simulink model "AEBS_A3X"  (Simulink 7.9)
settings: Solver=ode45  StartTime=0.0  StopTime=10.0  RelTol=1e-3
libraries: simulink x12
settings Model: Creator=fpt  LastModifiedBy=a55
settings HardwareCC: TargetIntDivRoundTo=Zero  TargetEndianess=LittleEndian  TargetHWDeviceType=MATLAB Host  ProdEqTarget=off
settings RTWCC: SystemTargetFile=rtwsfcnfmi.tlc  TemplateMakefile=rtwsfcnfmi_tmf  Description=S-function Target with Functional Model Interface (FMI)  ProcessScript=rtwsfcnfmi_make_rtw_hook
settings STFCustomTargetCC: CodeReplacementLibrary=ANSI_C  ModelReferenceCompliant=off  CompOptLevelCompliant=on  GeneratePreprocessorConditionals=Disable all  SystemTargetFile=rtwsfcnfmi.tlc
settings CustomProperty: Value=on

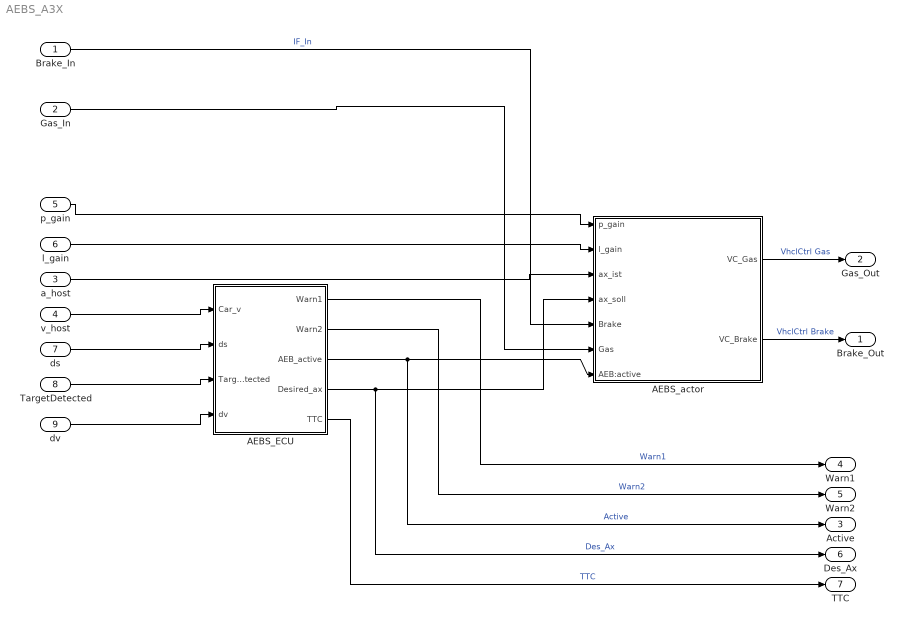
== system AEBS_A3X ==
  Brake_In : Inport  OutDataTypeStr=double
  Gas_In : Inport  Port=2  OutDataTypeStr=double
  a_host : Inport  Port=3  OutDataTypeStr=double
  v_host : Inport  Port=4  OutDataTypeStr=double
  p_gain : Inport  Port=5  OutDataTypeStr=double
  l_gain : Inport  Port=6  OutDataTypeStr=double
  ds : Inport  Port=7  OutDataTypeStr=double
  TargetDetected : Inport  Port=8  OutDataTypeStr=double
  dv : Inport  Port=9  OutDataTypeStr=double
  AEBS_ECU : Subsystem  Description=|
      | SL_REQ_010                                              
      | << Autonomous Emergency Braking ECU controller model>>
      | REQ_AB_01                    
      | R-0000057
  AEBS_actor : Subsystem  Description=|
      | SL_REQ_020                                              
      | << The Cruise control Speed Limit shall be implemented>>
      | REQ_AB_02                    
      | R-0000044                    
      | R-0000058                  
      | R-0000045
  Brake_Out : Outport  OutDataTypeStr=double
  Gas_Out : Outport  Port=2  OutDataTypeStr=double
  Active : Outport  Port=3  OutDataTypeStr=double
  Warn1 : Outport  Port=4  OutDataTypeStr=double
  Warn2 : Outport  Port=5  OutDataTypeStr=double
  Des_Ax : Outport  Port=6  OutDataTypeStr=double
  TTC : Outport  Port=7  OutDataTypeStr=double
  wires:
  AEBS_ECU/5(TTC) -> TTC/1  "TTC"
  AEBS_ECU/1(Warn1) -> Warn1/1  "Warn1"
  AEBS_ECU/2(Warn2) -> Warn2/1  "Warn2"
  AEBS_ECU/3(AEB_active) -> AEBS_actor/7(AEB:active), Active/1  "Active"
  AEBS_ECU/4(Desired_ax) -> AEBS_actor/4(ax_soll), Des_Ax/1  "Des_Ax"
  ds/1 -> AEBS_ECU/2(ds)
  v_host/1 -> AEBS_ECU/1(Car_v)
  a_host/1 -> AEBS_actor/3(ax_ist)
  p_gain/1 -> AEBS_actor/1(p_gain)
  Gas_In/1 -> AEBS_actor/6(Gas)
  TargetDetected/1 -> AEBS_ECU/3(TargetDetected)
  dv/1 -> AEBS_ECU/4(dv)
  l_gain/1 -> AEBS_actor/2(l_gain)
  Brake_In/1 -> AEBS_actor/5(Brake)  "IF_In"
  AEBS_actor/1(VC_Gas) -> Gas_Out/1  "VhclCtrl Gas"
  AEBS_actor/2(VC_Brake) -> Brake_Out/1  "VhclCtrl Brake"

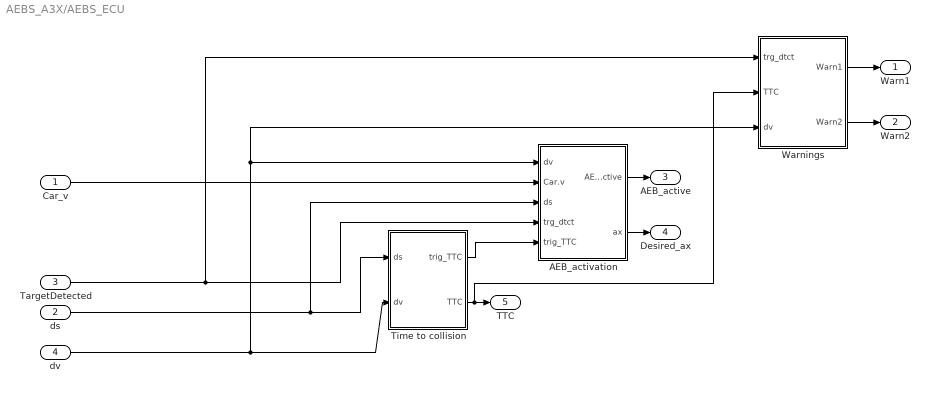
== system AEBS_A3X/AEBS_ECU ==
  Car_v : Inport  OutDataTypeStr=double
  ds : Inport  Port=2  OutDataTypeStr=double
  TargetDetected : Inport  Port=3  OutDataTypeStr=double
  dv : Inport  Port=4  OutDataTypeStr=double
  AEB_activation : Subsystem  Description=|
      | SL_REQ_011                                              
      | << The Cruise control Speed Limit shall be implemented>>
      | R-0000061                    
      | R-0000063
  Time to collision : Subsystem  Description=|
      | SL_REQ_013                                              
      | << The Cruise control Speed Limit shall be implemented>>
      | R-0000064                    
      | R-0000050                    
      | R-0000052
  Warnings : Subsystem  Description=|
      | SL_REQ_014                                              
      | << The Cruise control Speed Limit shall be implemented>>
      | R-0000048                    
      | R-0000050                    
      | R-0000052
  Warn1 : Outport  OutDataTypeStr=double
  Warn2 : Outport  Port=2  OutDataTypeStr=double
  AEB_active : Outport  Port=3  OutDataTypeStr=double
  Desired_ax : Outport  Port=4  OutDataTypeStr=double
  TTC : Outport  Port=5  OutDataTypeStr=double
  wires:
  TargetDetected/1 -> AEB_activation/4(trg_dtct), Warnings/1(trg_dtct)
  dv/1 -> AEB_activation/1(dv), Warnings/3(dv), Time to collision/2(dv)
  Time to collision/1(trig_TTC) -> AEB_activation/5(trig_TTC)
  AEB_activation/1(AEB_active) -> AEB_active/1
  Car_v/1 -> AEB_activation/2(Car.v)
  Warnings/1(Warn1) -> Warn1/1
  Warnings/2(Warn2) -> Warn2/1
  AEB_activation/2(ax) -> Desired_ax/1
  Time to collision/2(TTC) -> Warnings/2(TTC), TTC/1
  ds/1 -> AEB_activation/3(ds), Time to collision/1(ds)

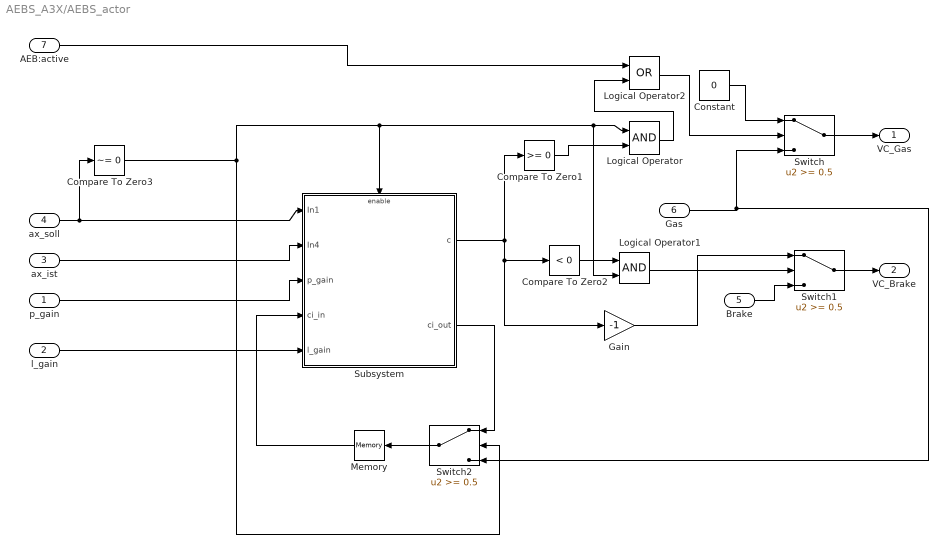
== system AEBS_A3X/AEBS_actor ==
  p_gain : Inport  OutDataTypeStr=double
  l_gain : Inport  Port=2  OutDataTypeStr=double
  ax_ist : Inport  Port=3  OutDataTypeStr=double
  ax_soll : Inport  Port=4  OutDataTypeStr=double
  Brake : Inport  Port=5  OutDataTypeStr=double
  Gas : Inport  Port=6  OutDataTypeStr=double
  AEB:active : Inport  Port=7  OutDataTypeStr=double
  Compare To Zero1 : simulink/Logic and Bit Operations/Compare To Zero  relop=>=  OutDataTypeStr=boolean
  Compare To Zero2 : simulink/Logic and Bit Operations/Compare To Zero  relop=<  OutDataTypeStr=boolean
  Compare To Zero3 : simulink/Logic and Bit Operations/Compare To Zero  relop=~=  OutDataTypeStr=boolean
  Constant : Constant  Value=0  OutDataTypeStr=double
  Gain : Gain  Gain=-1
  Logical Operator : Logic  AllPortsSameDT=off  OutDataTypeStr=boolean
  Logical Operator1 : Logic  AllPortsSameDT=off  OutDataTypeStr=boolean
  Logical Operator2 : Logic  Operator=OR  AllPortsSameDT=off  OutDataTypeStr=boolean
  Memory : Memory
  Subsystem : Subsystem
  Switch : Switch  Threshold=0.5  OutDataTypeStr=double
  Switch1 : Switch  Threshold=0.5  OutDataTypeStr=double
  Switch2 : Switch  Threshold=0.5  OutDataTypeStr=double
  VC_Gas : Outport  OutDataTypeStr=double
  VC_Brake : Outport  Port=2  OutDataTypeStr=double
  wires:
  ax_soll/1 -> Compare To Zero3/1, Subsystem/1(In1)
  ax_ist/1 -> Subsystem/2(In4)
  p_gain/1 -> Subsystem/3(p_gain)
  Switch/1 -> VC_Gas/1
  Switch1/1 -> VC_Brake/1
  Subsystem/1(c) -> Compare To Zero1/1, Compare To Zero2/1, Gain/1
  Compare To Zero1/1 -> Logical Operator/2
  Memory/1 -> Subsystem/4(ci_in)
  Subsystem/2(ci_out) -> Switch2/1
  Switch2/1 -> Memory/1
  Logical Operator1/1 -> Switch1/2
  Compare To Zero2/1 -> Logical Operator1/1
  Brake/1 -> Switch1/3
  Gain/1 -> Switch1/1
  Compare To Zero3/1 -> Logical Operator1/2, Logical Operator/1, Subsystem/Enable, Switch2/2
  Constant/1 -> Switch/1
  Gas/1 -> Switch2/3, Switch/3
  Logical Operator2/1 -> Switch/2
  Logical Operator/1 -> Logical Operator2/2
  AEB:active/1 -> Logical Operator2/1
  l_gain/1 -> Subsystem/5(l_gain)

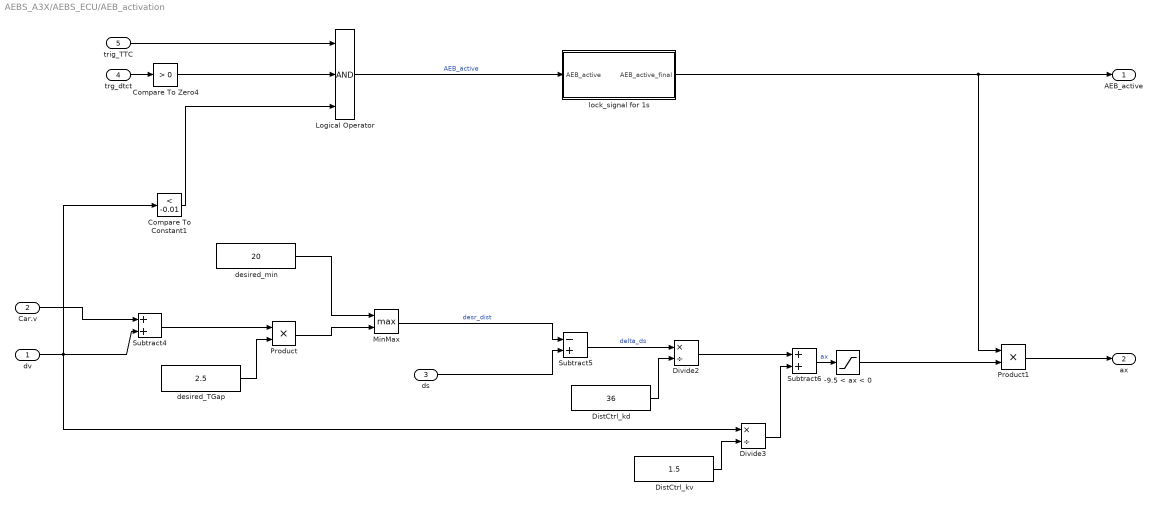
== system AEBS_A3X/AEBS_ECU/AEB_activation ==
  dv : Inport  OutDataTypeStr=double
  Car.v : Inport  Port=2  OutDataTypeStr=double
  ds : Inport  Port=3  OutDataTypeStr=double
  trg_dtct : Inport  Port=4  OutDataTypeStr=double
  trig_TTC : Inport  Description=|  Port=5  OutDataTypeStr=double
      | SL_REQ_111                                              
      | << The Cruise control Speed Limit shall be implemented>>
      | R-0000062
  -9.5 < ax < 0 : Saturate  UpperLimit=0  LowerLimit=-9.5
  Compare To Constant1 : simulink/Logic and Bit Operations/Compare To Constant  relop=<  const=-0.01  OutDataTypeStr=uint8
  Compare To Zero4 : simulink/Logic and Bit Operations/Compare To Zero  relop=>  OutDataTypeStr=uint8
  DistCtrl_kd : Constant  Value=36  OutDataTypeStr=double
  DistCtrl_kv : Constant  Value=1.5  OutDataTypeStr=double
  Divide2 : Product  Inputs=*/
  Divide3 : Product  Inputs=*/
  Logical Operator : Logic  Inputs=3  AllPortsSameDT=off  OutDataTypeStr=boolean
  MinMax : MinMax  Function=max  Inputs=2
  Product : Product  RndMeth=Zero
  Product1 : Product  RndMeth=Zero
  Subtract4 : Sum
  Subtract5 : Sum  Inputs=-+
  Subtract6 : Sum
  desired_TGap : Constant  Value=2.5  OutDataTypeStr=double
  desired_min : Constant  Value=20  OutDataTypeStr=double
  lock_signal for 1s : Subsystem  Description=|
      | SL_REQ_012                                              
      | << The Cruise control Speed Limit shall be implemented>>
      | R-0000062                  
      | R-0000050                    
      | R-0000052
  AEB_active : Outport  OutDataTypeStr=double
  ax : Outport  Port=2  OutDataTypeStr=double
  wires:
  dv/1 -> Subtract4/2, Divide3/1, Compare To Constant1/1
  Car.v/1 -> Subtract4/1
  desired_min/1 -> MinMax/1
  Subtract4/1 -> Product/1
  desired_TGap/1 -> Product/2
  Product/1 -> MinMax/2
  MinMax/1 -> Subtract5/1  "desr_dist"
  ds/1 -> Subtract5/2
  Subtract5/1 -> Divide2/1  "delta_ds"
  DistCtrl_kd/1 -> Divide2/2
  DistCtrl_kv/1 -> Divide3/2
  Divide2/1 -> Subtract6/1
  Divide3/1 -> Subtract6/2
  Subtract6/1 -> -9.5 < ax < 0/1  "ax"
  trg_dtct/1 -> Compare To Zero4/1
  Compare To Zero4/1 -> Logical Operator/2
  Compare To Constant1/1 -> Logical Operator/3
  trig_TTC/1 -> Logical Operator/1
  -9.5 < ax < 0/1 -> Product1/2
  Product1/1 -> ax/1
  lock_signal for 1s/1(AEB_active_final) -> AEB_active/1, Product1/1
  Logical Operator/1 -> lock_signal for 1s/1(AEB_active)  "AEB_active"

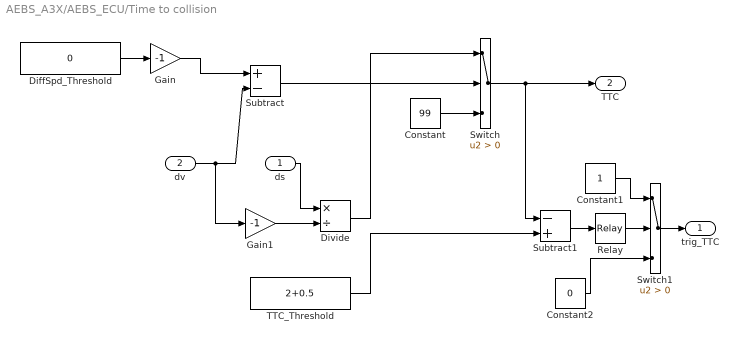
== system AEBS_A3X/AEBS_ECU/Time to collision ==
  ds : Inport  OutDataTypeStr=double
  dv : Inport  Port=2  OutDataTypeStr=double
  Constant : Constant  Value=99  OutDataTypeStr=double
  Constant1 : Constant  OutDataTypeStr=double
  Constant2 : Constant  Value=0  OutDataTypeStr=double
  DiffSpd_Threshold : Constant  Value=0  OutDataTypeStr=double
  Divide : Product  Inputs=*/
  Gain : Gain  Gain=-1
  Gain1 : Gain  Gain=-1
  Relay : Relay  OnSwitchValue=0.5  OffSwitchValue=0
  Subtract : Sum  Inputs=+-
  Subtract1 : Sum  Inputs=-+
  Switch : Switch  Criteria=u2 > Threshold  OutDataTypeStr=double
  Switch1 : Switch  Criteria=u2 > Threshold  OutDataTypeStr=double
  TTC_Threshold : Constant  Value=2+0.5  OutDataTypeStr=double
  trig_TTC : Outport  OutDataTypeStr=double
  TTC : Outport  Port=2  OutDataTypeStr=double
  wires:
  dv/1 -> Subtract/2, Gain1/1
  DiffSpd_Threshold/1 -> Gain/1
  Gain/1 -> Subtract/1
  Gain1/1 -> Divide/2
  Divide/1 -> Switch/1
  TTC_Threshold/1 -> Subtract1/2
  Subtract/1 -> Switch/2
  Constant/1 -> Switch/3
  Switch/1 -> Subtract1/1, TTC/1
  Subtract1/1 -> Relay/1
  Constant1/1 -> Switch1/1
  Constant2/1 -> Switch1/3
  Switch1/1 -> trig_TTC/1
  ds/1 -> Divide/1
  Relay/1 -> Switch1/2

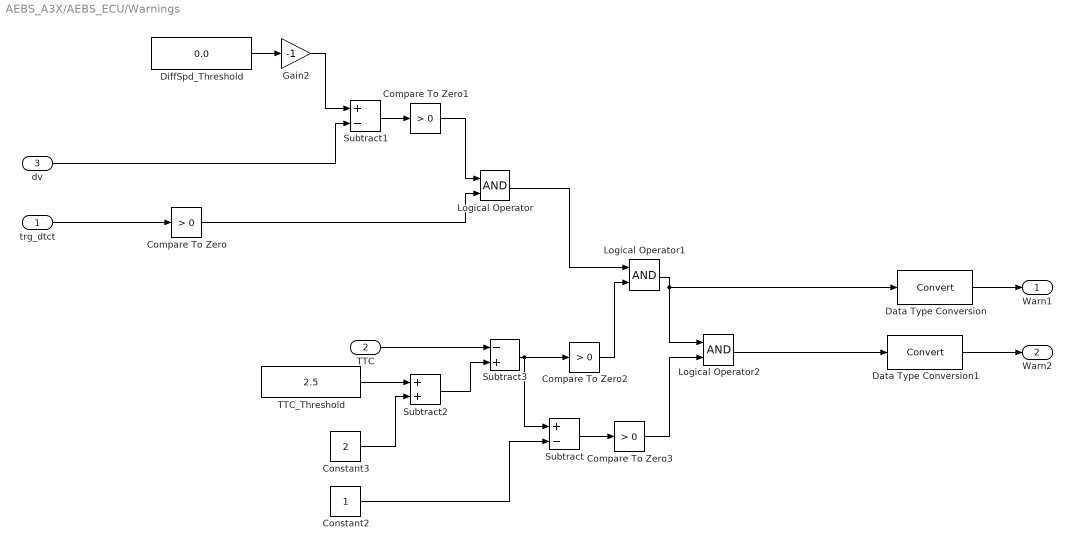
== system AEBS_A3X/AEBS_ECU/Warnings ==
  trg_dtct : Inport  OutDataTypeStr=double
  TTC : Inport  Port=2  OutDataTypeStr=double
  dv : Inport  Port=3  OutDataTypeStr=double
  Compare To Zero{,1..3} (4 alike) : simulink/Logic and Bit Operations/Compare To Zero  relop=>  OutDataTypeStr=uint8
  Constant2 : Constant  OutDataTypeStr=double
  Constant3 : Constant  Value=2  OutDataTypeStr=double
  Data Type Conversion : DataTypeConversion
  Data Type Conversion1 : DataTypeConversion
  DiffSpd_Threshold : Constant  Value=0.0  OutDataTypeStr=double
  Gain2 : Gain  Gain=-1
  Logical Operator : Logic  AllPortsSameDT=off  OutDataTypeStr=boolean
  Logical Operator1 : Logic  AllPortsSameDT=off  OutDataTypeStr=boolean
  Logical Operator2 : Logic  AllPortsSameDT=off  OutDataTypeStr=boolean
  Subtract : Sum  Inputs=+-
  Subtract1 : Sum  Inputs=+-
  Subtract2 : Sum
  Subtract3 : Sum  Inputs=-+
  TTC_Threshold : Constant  Value=2.5  OutDataTypeStr=double
  Warn1 : Outport  OutDataTypeStr=double
  Warn2 : Outport  Port=2  OutDataTypeStr=double
  wires:
  dv/1 -> Subtract1/2
  trg_dtct/1 -> Compare To Zero/1
  DiffSpd_Threshold/1 -> Gain2/1
  Gain2/1 -> Subtract1/1
  Subtract1/1 -> Compare To Zero1/1
  Compare To Zero1/1 -> Logical Operator/1
  Compare To Zero/1 -> Logical Operator/2
  TTC_Threshold/1 -> Subtract2/1
  Constant3/1 -> Subtract2/2
  Subtract2/1 -> Subtract3/2
  Subtract3/1 -> Compare To Zero2/1, Subtract/1
  Logical Operator/1 -> Logical Operator1/1
  Compare To Zero2/1 -> Logical Operator1/2
  Subtract/1 -> Compare To Zero3/1
  Constant2/1 -> Subtract/2
  Compare To Zero3/1 -> Logical Operator2/2
  Logical Operator1/1 -> Data Type Conversion/1, Logical Operator2/1
  Logical Operator2/1 -> Data Type Conversion1/1
  Data Type Conversion/1 -> Warn1/1
  Data Type Conversion1/1 -> Warn2/1
  TTC/1 -> Subtract3/1

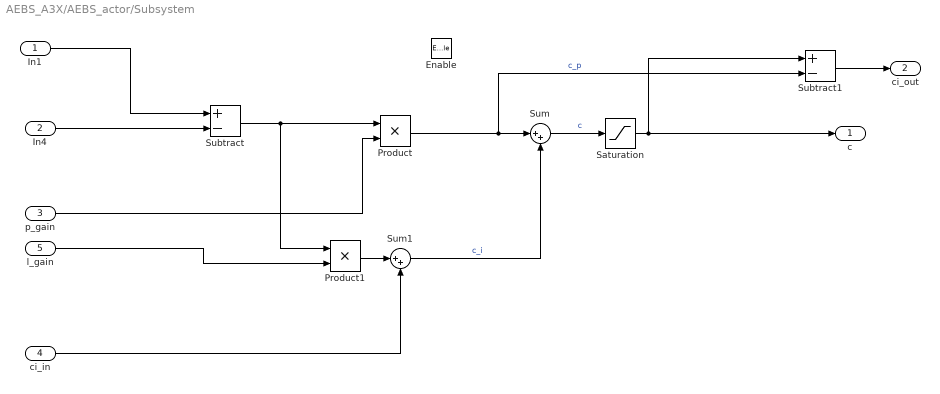
== system AEBS_A3X/AEBS_actor/Subsystem ==
  In1 : Inport  OutDataTypeStr=double
  In4 : Inport  Port=2  OutDataTypeStr=double
  p_gain : Inport  Port=3  OutDataTypeStr=double
  ci_in : Inport  Port=4  OutDataTypeStr=double
  l_gain : Inport  Port=5  OutDataTypeStr=double
  Enable : EnablePort
  Product : Product  RndMeth=Zero
  Product1 : Product  RndMeth=Zero
  Saturation : Saturate  UpperLimit=1  LowerLimit=-1
  Subtract : Sum  Inputs=+-
  Subtract1 : Sum  Inputs=+-
  Sum : Sum  Inputs=|++
  Sum1 : Sum  Inputs=|++
  c : Outport  OutDataTypeStr=double
  ci_out : Outport  Port=2  OutDataTypeStr=double
  wires:
  In4/1 -> Subtract/2
  In1/1 -> Subtract/1
  Subtract/1 -> Product1/1, Product/1
  p_gain/1 -> Product/2
  Product/1 -> Subtract1/2, Sum/1  "c_p"
  Sum1/1 -> Sum/2  "c_i"
  l_gain/1 -> Product1/2
  Product1/1 -> Sum1/1
  Sum/1 -> Saturation/1  "c"
  Saturation/1 -> Subtract1/1, c/1
  Subtract1/1 -> ci_out/1
  ci_in/1 -> Sum1/2

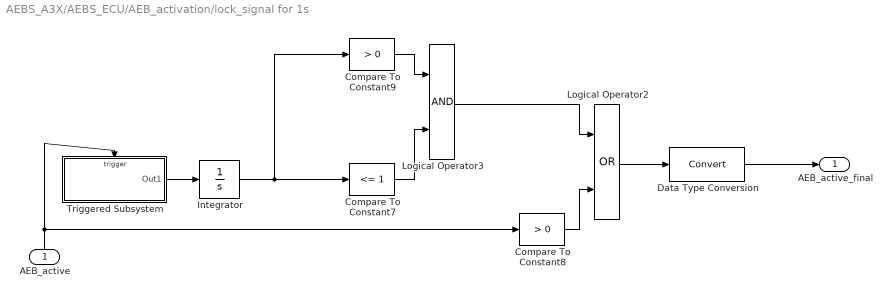
== system AEBS_A3X/AEBS_ECU/AEB_activation/lock_signal for 1s ==
  AEB_active : Inport  OutDataTypeStr=boolean
  Compare To Constant7 : simulink/Logic and Bit Operations/Compare To Constant  relop=<=  const=1  OutDataTypeStr=uint8
  Compare To Constant8 : simulink/Logic and Bit Operations/Compare To Constant  relop=>  const=0  OutDataTypeStr=uint8
  Compare To Constant9 : simulink/Logic and Bit Operations/Compare To Constant  relop=>  const=0  OutDataTypeStr=uint8
  Data Type Conversion : DataTypeConversion
  Integrator : Integrator
  Logical Operator2 : Logic  Operator=OR  AllPortsSameDT=off  OutDataTypeStr=boolean
  Logical Operator3 : Logic  AllPortsSameDT=off  OutDataTypeStr=boolean
  Triggered Subsystem : Subsystem  TreatAsAtomicUnit=on
  AEB_active_final : Outport  OutDataTypeStr=double
  wires:
  AEB_active/1 -> Compare To Constant8/1, Triggered Subsystem/Trigger
  Integrator/1 -> Compare To Constant7/1, Compare To Constant9/1
  Triggered Subsystem/1(Out1) -> Integrator/1
  Compare To Constant8/1 -> Logical Operator2/2
  Compare To Constant9/1 -> Logical Operator3/1
  Compare To Constant7/1 -> Logical Operator3/2
  Logical Operator3/1 -> Logical Operator2/1
  Logical Operator2/1 -> Data Type Conversion/1
  Data Type Conversion/1 -> AEB_active_final/1

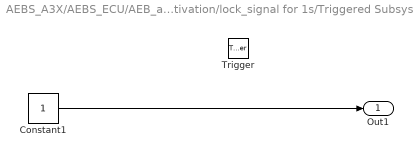
== system AEBS_A3X/AEBS_ECU/AEB_activation/lock_signal for 1s/Triggered Subsystem ==
  Trigger : TriggerPort  TriggerType=falling
  Constant1 : Constant  OutDataTypeStr=double
  Out1 : Outport  OutDataTypeStr=double  InitialOutput=0
  wires:
  Constant1/1 -> Out1/1
